simulink model "rx80211a3l"  (R2016a)
settings: Solver=FixedStepDiscrete  SolverMode=SingleTasking  StartTime=0.0  StopTime=46*tpf  RelTol=1e-3
PreLoadFcn:
  | [srx, str, ffv, stx, stb, spi, spl, spq, ntf, cdi, cds] = rx80211a_r0();
InitFcn:
  | if ~exist('srx','var')
  | [srx, str, ffv, stx, stb, spi, spl, spq, ntf, cdi, cds] = rx80211a_r0();
  | end
  | bitrate = 6e6; % 6 Mbits per second
  | crf = 2; % constant redundancy factor (from conv enc)
  | nepsc = 16; % #empty+pilot subcarriers
  | ncps = 16; % #cyclic prefix samples
  | ndbpf = 24; % #data bits per frame
  | ncbpf = ndbpf * crf; % #coded bits per frame
  | nscpf = ncbpf + nepsc; % #subcarriers per frame
  | nspf = nscpf + 16; % #samples per frame
  | tps = 1e-5; %tpf/nspf; % sample time
  | tpf = tps*nspf; %ndbpf/bitrate; % frame time
undefined symbols (not defined in the file): cds, ntf, srx
libraries: hdlsllib x34, simulink x17, dspxfrm3 x1, dspstat3 x1, commdigbbndpm3 x1, commcnvcod2 x1
settings Model: Creator=wchen  LastModifiedBy=bdroz
settings DataIOCC: LimitDataPoints=on  SaveFormat=Array  SaveOutput=off  SignalLogging=off  SaveTime=off
settings OptimizationCC: BlockReduction=off  ConditionallyExecuteInputs=off  DefaultParameterBehavior=Inlined  ExpressionDepthLimit=2147483647
settings DebuggingCC: AlgebraicLoopMsg=error  UnderspecifiedInitializationDetection=Classic  MergeDetectMultiDrivingBlocksExec=none  SolverPrmCheckMsg=warning  SingleTaskRateTransMsg=error  IntegerOverflowMsg=none  ParameterPrecisionLossMsg=none  AllowSymbolicDim=off  StateNameClashWarn=warning
settings HardwareCC: ProdBitPerPointer=32  ProdLargestAtomicFloat=None  ProdIntDivRoundTo=Undefined  ProdEndianess=Unspecified  ProdWordSize=32  ProdHWDeviceType=ASIC/FPGA->ASIC/FPGA  TargetBitPerPointer=64  TargetLongLongMode=on  TargetIntDivRoundTo=Zero  TargetEndianess=LittleEndian  TargetWordSize=64  TargetHWDeviceType=MATLAB Host  ProdEqTarget=off
settings ModelReferenceCC: PropagateSignalLabelsOutOfModel=off
settings ConfigComp: CovModelRefEnable=Off

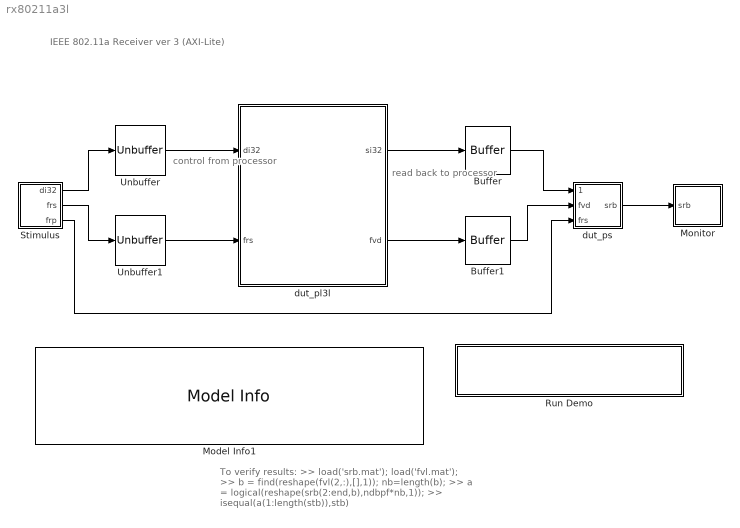
== system rx80211a3l ==
  note: control from
      | processor
  note: IEEE 802.11a Receiver ver 3 (AXI-Lite)
  note: read back to
      | processor
  note: To verify results:
      | >> load('srb.mat'); load('fvl.mat');
      | >> b = find(reshape(fvl(2,:),[],1)); nb=length(b);
      | >> a = logical(reshape(srb(2:end,b),ndbpf*nb,1));
      | >> isequal(a(1:length(stb)),stb)
  Buffer : Buffer  N=nspf  TreatMby1Signals=One channel  OutputFrames=off
  Buffer1 : Buffer  N=nspf  TreatMby1Signals=One channel  OutputFrames=off
  Model Info1 : simulink/Model-Wide Utilities/Model Info  Frame=on  DisplayStringWithTags=|  HorizontalTextAlignment=Left  LeftAlignmentValue=0.02  SourceBlockDiagram=rx80211a3l  TagMaxNumber=20
      | This example shows how to use HDL Workflow Advisor to 
      | generate a custom IP core which blink LEDs on FPGA board.
      | 
      | In MATLAB, type the following:
      |   hdladvisor('rx80211a3l/dut_pl3l')
  Monitor : Subsystem  TreatAsAtomicUnit=on
  Run Demo : Subsystem
      settings: OpenFcn=hdladvisor([bdroot, '/dut_pl'])
      mask Display: disp('Launch HDL Workflow Advisor')
  Stimulus : Subsystem
  Unbuffer : Unbuffer  SampleBasedProcessing=Same as frame based
  Unbuffer1 : Unbuffer  SampleBasedProcessing=Same as frame based
  dut_pl3l : Subsystem  TreatAsAtomicUnit=on
  dut_ps : Subsystem
  wires:
  Stimulus/1(di32) -> Unbuffer/1
  dut_pl3l/1(si32) -> Buffer/1
  Unbuffer/1 -> dut_pl3l/1(di32)
  Buffer/1 -> dut_ps/1(si32)
  dut_ps/1(srb) -> Monitor/1(srb)
  Stimulus/2(frs) -> Unbuffer1/1
  Unbuffer1/1 -> dut_pl3l/2(frs)
  dut_pl3l/2(fvd) -> Buffer1/1
  Buffer1/1 -> dut_ps/2(fvd)
  Stimulus/3(frp) -> dut_ps/3(frs)

== system rx80211a3l/Monitor ==
  srb : Inport
  Compare To Constant : simulink/Logic and Bit Operations/Compare To Constant  relop=>  const=uint16(0)  OutDataTypeStr=boolean
  Counter Free-Running : simulink/Sources/Counter Free-Running  NumBits=16  tsamp=tpf
  unpack_int32_into_bool24 : Subsystem
  write_srb_to_file1 : Subsystem
  wires:
  Counter Free-Running/1 -> Compare To Constant/1
  Compare To Constant/1 -> write_srb_to_file1/Enable
  unpack_int32_into_bool24/1(stx) -> write_srb_to_file1/1(srb)
  unpack_int32_into_bool24/2(fvd) -> write_srb_to_file1/2(fvl)
  srb/1 -> unpack_int32_into_bool24/1(di32)

== system rx80211a3l/Run Demo ==

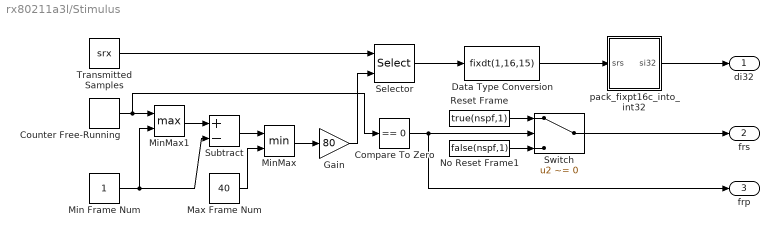
== system rx80211a3l/Stimulus ==
  Compare To Zero : simulink/Logic and Bit Operations/Compare To Zero  relop===  OutDataTypeStr=boolean
  Counter Free-Running : simulink/Sources/Counter Free-Running  NumBits=16  tsamp=tpf
  Data Type Conversion : DataTypeConversion  OutDataTypeStr=fixdt(1,16,15)
  Gain : Gain  Gain=80  OutDataTypeStr=uint16
  Max Frame Num : Constant  Value=40  OutDataTypeStr=uint16  SampleTime=tpf
  Min Frame Num : Constant  OutDataTypeStr=uint16  SampleTime=tpf
  MinMax : MinMax  Inputs=2
  MinMax1 : MinMax  Function=max  Inputs=2
  No Reset Frame1 : Constant  Value=false(nspf,1)  OutDataTypeStr=boolean  SampleTime=tpf
  Reset Frame : Constant  Value=true(nspf,1)  OutDataTypeStr=boolean  SampleTime=tpf
  Selector : Selector  IndexMode=Zero-based  InputPortWidth=3280  IndexOptions=Starting index (port)  Indices=[1 3]  OutputSizes=80
  Subtract : Sum  Inputs=+-
  Switch : Switch  Criteria=u2 ~= 0
  Transmitted Samples : Constant  Value=srx  SampleTime=tpf
  pack_fixpt16c_into_int32 : Subsystem
  di32 : Outport
  frs : Outport  Port=2
  frp : Outport  Port=3
  wires:
  Counter Free-Running/1 -> Compare To Zero/1, MinMax1/1
  Max Frame Num/1 -> MinMax/2
  MinMax/1 -> Gain/1
  Transmitted Samples/1 -> Selector/1
  Gain/1 -> Selector/2
  Selector/1 -> Data Type Conversion/1
  Data Type Conversion/1 -> pack_fixpt16c_into_int32/1(srs)
  pack_fixpt16c_into_int32/1(si32) -> di32/1
  Min Frame Num/1 -> MinMax1/2, Subtract/2
  Subtract/1 -> MinMax/1
  MinMax1/1 -> Subtract/1
  Compare To Zero/1 -> frp/1, Switch/2
  Switch/1 -> frs/1
  Reset Frame/1 -> Switch/1
  No Reset Frame1/1 -> Switch/3

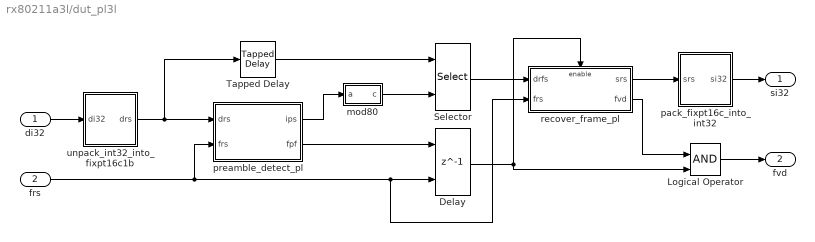
== system rx80211a3l/dut_pl3l ==
  di32 : Inport  OutDataTypeStr=uint32
  frs : Inport  Port=2  OutDataTypeStr=boolean
  Delay : Delay  DelayLength=1  InitialCondition=false  ExternalReset=Level  SampleTime=tps
      settings: InputPortMap=u0,r5
  Logical Operator : Logic  IconShape=distinctive  AllPortsSameDT=off  OutDataTypeStr=boolean
  Selector : Selector  IndexMode=Zero-based  InputPortWidth=80  IndexOptions=Starting index (port)  Indices=[1 3]  OutputSizes=1
  Tapped Delay : simulink/Discrete/Tapped Delay  vinit=complex(0.0)  samptime=tps  NumDelays=79  DelayOrder=Oldest  includeCurrent=on
  mod80 : Subsystem
  pack_fixpt16c_into_int32 : Subsystem
  preamble_detect_pl : Subsystem
  recover_frame_pl : Subsystem  TreatAsAtomicUnit=on
  unpack_int32_into_fixpt16c1b : Subsystem
  si32 : Outport
  fvd : Outport  Port=2
  wires:
  di32/1 -> unpack_int32_into_fixpt16c1b/1(di32)
  unpack_int32_into_fixpt16c1b/1(drs) -> Tapped Delay/1, preamble_detect_pl/1(drs)
  preamble_detect_pl/2(fpf) -> Delay/1
  recover_frame_pl/1(srs) -> pack_fixpt16c_into_int32/1(srs)
  Tapped Delay/1 -> Selector/1
  preamble_detect_pl/1(ips) -> mod80/1(a)
  Selector/1 -> recover_frame_pl/1(drfs)
  mod80/1(c) -> Selector/2
  Delay/1 -> recover_frame_pl/Enable, Logical Operator/2
  frs/1 -> preamble_detect_pl/2(frs), recover_frame_pl/2(frs), Delay/2
  pack_fixpt16c_into_int32/1(si32) -> si32/1
  Logical Operator/1 -> fvd/1
  recover_frame_pl/2(fvd) -> Logical Operator/1

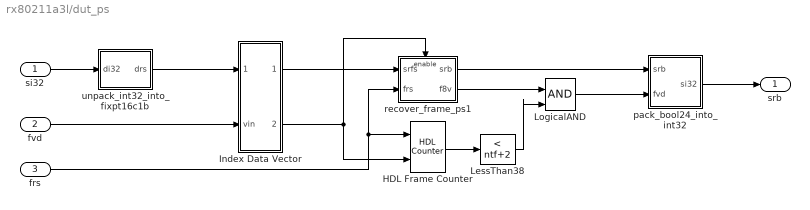
== system rx80211a3l/dut_ps ==
  si32 : Inport
  fvd : Inport  Port=2
  frs : Inport  Port=3
  HDL Frame Counter : hdlsllib/HDL Operations/HDL Counter  CountType=Free running  CountInit=0  CountStep=1  CountMax=25  CountFromType=Initial value  CountFrom=0  CountResetPort=on  CountLoadPort=off  CountEnbPort=on  CountDirPort=off  CountDataType=Unsigned  CountWordLen=8  CountFracLen=0  CountSampTime=1
  Index Data Vector : Subsystem
  LessThan38 : simulink/Logic and Bit Operations/Compare To Constant  relop=<  const=ntf+2  OutDataTypeStr=boolean
  LogicalAND : Logic  IconShape=distinctive  AllPortsSameDT=off  OutDataTypeStr=boolean
  pack_bool24_into_int32 : Subsystem
  recover_frame_ps1 : Subsystem  TreatAsAtomicUnit=on
  unpack_int32_into_fixpt16c1b : Subsystem
  srb : Outport
  wires:
  recover_frame_ps1/1(srb) -> pack_bool24_into_int32/1(srb)
  pack_bool24_into_int32/1(si32) -> srb/1
  frs/1 -> recover_frame_ps1/2(frs), HDL Frame Counter/1
  HDL Frame Counter/1 -> LessThan38/1
  LessThan38/1 -> LogicalAND/2
  LogicalAND/1 -> pack_bool24_into_int32/2(fvd)
  recover_frame_ps1/2(f8v) -> LogicalAND/1
  si32/1 -> unpack_int32_into_fixpt16c1b/1(di32)
  Index Data Vector/2(vout) -> recover_frame_ps1/Enable, HDL Frame Counter/2
  fvd/1 -> Index Data Vector/2(vin)
  unpack_int32_into_fixpt16c1b/1(drs) -> Index Data Vector/1(din)
  Index Data Vector/1(dout) -> recover_frame_ps1/1(srfs)

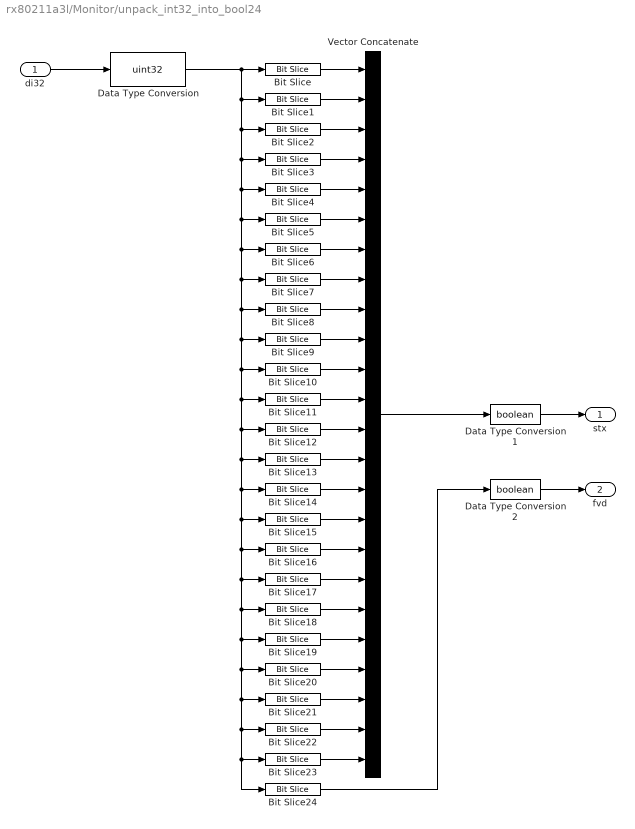
== system rx80211a3l/Monitor/unpack_int32_into_bool24 ==
  di32 : Inport
  Bit Slice : hdlsllib/HDL Operations/Bit Slice  lidx=31  ridx=31
      settings: AttributesFormatString=%<lidx>
  Bit Slice1 : hdlsllib/HDL Operations/Bit Slice  lidx=30  ridx=30
      settings: AttributesFormatString=%<lidx>
  Bit Slice10 : hdlsllib/HDL Operations/Bit Slice  lidx=21  ridx=21
      settings: AttributesFormatString=%<lidx>
  Bit Slice11 : hdlsllib/HDL Operations/Bit Slice  lidx=20  ridx=20
      settings: AttributesFormatString=%<lidx>
  Bit Slice12 : hdlsllib/HDL Operations/Bit Slice  lidx=19  ridx=19
      settings: AttributesFormatString=%<lidx>
  Bit Slice13 : hdlsllib/HDL Operations/Bit Slice  lidx=18  ridx=18
      settings: AttributesFormatString=%<lidx>
  Bit Slice14 : hdlsllib/HDL Operations/Bit Slice  lidx=17  ridx=17
      settings: AttributesFormatString=%<lidx>
  Bit Slice15 : hdlsllib/HDL Operations/Bit Slice  lidx=16  ridx=16
      settings: AttributesFormatString=%<lidx>
  Bit Slice16 : hdlsllib/HDL Operations/Bit Slice  lidx=15  ridx=15
      settings: AttributesFormatString=%<lidx>
  Bit Slice17 : hdlsllib/HDL Operations/Bit Slice  lidx=14  ridx=14
      settings: AttributesFormatString=%<lidx>
  Bit Slice18 : hdlsllib/HDL Operations/Bit Slice  lidx=13  ridx=13
      settings: AttributesFormatString=%<lidx>
  Bit Slice19 : hdlsllib/HDL Operations/Bit Slice  lidx=12  ridx=12
      settings: AttributesFormatString=%<lidx>
  Bit Slice2 : hdlsllib/HDL Operations/Bit Slice  lidx=29  ridx=29
      settings: AttributesFormatString=%<lidx>
  Bit Slice20 : hdlsllib/HDL Operations/Bit Slice  lidx=11  ridx=11
      settings: AttributesFormatString=%<lidx>
  Bit Slice21 : hdlsllib/HDL Operations/Bit Slice  lidx=10  ridx=10
      settings: AttributesFormatString=%<lidx>
  Bit Slice22 : hdlsllib/HDL Operations/Bit Slice  lidx=9  ridx=9
      settings: AttributesFormatString=%<lidx>
  Bit Slice23 : hdlsllib/HDL Operations/Bit Slice  lidx=8  ridx=8
      settings: AttributesFormatString=%<lidx>
  Bit Slice24 : hdlsllib/HDL Operations/Bit Slice  lidx=7  ridx=7
      settings: AttributesFormatString=%<lidx>
  Bit Slice3 : hdlsllib/HDL Operations/Bit Slice  lidx=28  ridx=28
      settings: AttributesFormatString=%<lidx>
  Bit Slice4 : hdlsllib/HDL Operations/Bit Slice  lidx=27  ridx=27
      settings: AttributesFormatString=%<lidx>
  Bit Slice5 : hdlsllib/HDL Operations/Bit Slice  lidx=26  ridx=26
      settings: AttributesFormatString=%<lidx>
  Bit Slice6 : hdlsllib/HDL Operations/Bit Slice  lidx=25  ridx=25
      settings: AttributesFormatString=%<lidx>
  Bit Slice7 : hdlsllib/HDL Operations/Bit Slice  lidx=24  ridx=24
      settings: AttributesFormatString=%<lidx>
  Bit Slice8 : hdlsllib/HDL Operations/Bit Slice  lidx=23  ridx=23
      settings: AttributesFormatString=%<lidx>
  Bit Slice9 : hdlsllib/HDL Operations/Bit Slice  lidx=22  ridx=22
      settings: AttributesFormatString=%<lidx>
  Data Type Conversion : DataTypeConversion  OutDataTypeStr=uint32  ConvertRealWorld=Stored Integer (SI)
  Data Type Conversion1 : DataTypeConversion  OutDataTypeStr=boolean
  Data Type Conversion2 : DataTypeConversion  OutDataTypeStr=boolean
  Vector Concatenate : Concatenate  NumInputs=24
  stx : Outport
  fvd : Outport  Port=2
  wires:
  di32/1 -> Data Type Conversion/1
  Vector Concatenate/1 -> Data Type Conversion1/1
  Bit Slice24/1 -> Data Type Conversion2/1
  Data Type Conversion/1 -> Bit Slice1/1, Bit Slice2/1, Bit Slice3/1, Bit Slice4/1, Bit Slice5/1, Bit Slice7/1, Bit Slice8/1, Bit Slice9/1, Bit Slice11/1, Bit Slice12/1, Bit Slice13/1, Bit Slice15/1, Bit Slice17/1, Bit Slice18/1, Bit Slice19/1, Bit Slice20/1, Bit Slice21/1, Bit Slice24/1, Bit Slice23/1, Bit Slice22/1, Bit Slice16/1, Bit Slice14/1, Bit Slice10/1, Bit Slice6/1, Bit Slice/1
  Bit Slice23/1 -> Vector Concatenate/24
  Bit Slice22/1 -> Vector Concatenate/23
  Bit Slice21/1 -> Vector Concatenate/22
  Bit Slice20/1 -> Vector Concatenate/21
  Bit Slice19/1 -> Vector Concatenate/20
  Bit Slice18/1 -> Vector Concatenate/19
  Bit Slice17/1 -> Vector Concatenate/18
  Bit Slice16/1 -> Vector Concatenate/17
  Bit Slice15/1 -> Vector Concatenate/16
  Bit Slice14/1 -> Vector Concatenate/15
  Bit Slice13/1 -> Vector Concatenate/14
  Bit Slice12/1 -> Vector Concatenate/13
  Bit Slice11/1 -> Vector Concatenate/12
  Bit Slice10/1 -> Vector Concatenate/11
  Bit Slice9/1 -> Vector Concatenate/10
  Bit Slice8/1 -> Vector Concatenate/9
  Bit Slice7/1 -> Vector Concatenate/8
  Bit Slice6/1 -> Vector Concatenate/7
  Bit Slice5/1 -> Vector Concatenate/6
  Bit Slice4/1 -> Vector Concatenate/5
  Bit Slice3/1 -> Vector Concatenate/4
  Bit Slice2/1 -> Vector Concatenate/3
  Bit Slice1/1 -> Vector Concatenate/2
  Bit Slice/1 -> Vector Concatenate/1
  Data Type Conversion1/1 -> stx/1
  Data Type Conversion2/1 -> fvd/1

== system rx80211a3l/Monitor/write_srb_to_file1 ==
  srb : Inport
  fvl : Inport  Port=2
  Enable : EnablePort
  Data Type Conversion : DataTypeConversion  OutDataTypeStr=double
  Data Type Conversion1 : DataTypeConversion  OutDataTypeStr=double
  To File : ToFile  Filename=srb.mat  MatrixName=srb  SampleTime=tpf
  To File1 : ToFile  Filename=fvl.mat  MatrixName=fvl  SampleTime=tpf
  wires:
  fvl/1 -> Data Type Conversion1/1
  Data Type Conversion1/1 -> To File1/1
  srb/1 -> Data Type Conversion/1
  Data Type Conversion/1 -> To File/1

== system rx80211a3l/Stimulus/pack_fixpt16c_into_int32 ==
  srs : Inport
  Bit Concat : hdlsllib/HDL Operations/Bit Concat  numInputs=2
  Complex to Real-Imag : ComplexToRealImag
  si32 : Outport
  wires:
  srs/1 -> Complex to Real-Imag/1
  Complex to Real-Imag/1 -> Bit Concat/1
  Bit Concat/1 -> si32/1
  Complex to Real-Imag/2 -> Bit Concat/2

== system rx80211a3l/dut_pl3l/mod80 ==
  a : Inport
  Constant80 : Constant  Value=uint8(80)  OutDataTypeStr=uint8  SampleTime=tps
  Divide : Product  Inputs=*/  SaturateOnIntegerOverflow=on  RndMeth=Zero
  Product : Product  OutDataTypeStr=uint8
  Subtract : Sum  Inputs=+-  OutDataTypeStr=uint8
  c : Outport
  wires:
  a/1 -> Subtract/1, Divide/1  "a"
  Constant80/1 -> Product/2, Divide/2  "b"
  Divide/1 -> Product/1
  Product/1 -> Subtract/2
  Subtract/1 -> c/1  "c"

== system rx80211a3l/dut_pl3l/pack_fixpt16c_into_int32 ==
  srs : Inport
  Bit Concat : hdlsllib/HDL Operations/Bit Concat  numInputs=2
  Complex to Real-Imag : ComplexToRealImag
  si32 : Outport
  wires:
  srs/1 -> Complex to Real-Imag/1
  Complex to Real-Imag/1 -> Bit Concat/1
  Bit Concat/1 -> si32/1
  Complex to Real-Imag/2 -> Bit Concat/2

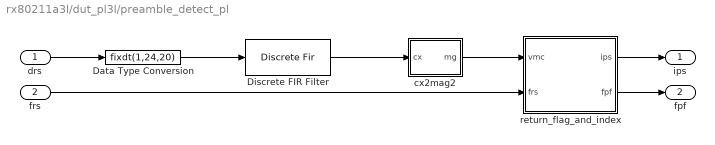
== system rx80211a3l/dut_pl3l/preamble_detect_pl ==
  drs : Inport
  frs : Inport  Port=2
  Data Type Conversion : DataTypeConversion  OutDataTypeStr=fixdt(1,24,20)
      settings: AttributesFormatString=%<OutDataTypeStr>
  Discrete FIR Filter : DiscreteFir  Coefficients=spl(end:-1:1)'  InitialStates=complex(0.0)  SampleTime=tps  CoefDataTypeStr=fixdt(1,24,20)  ProductDataTypeStr=fixdt(1,24,20)  AccumDataTypeStr=fixdt(1,24,20)  OutDataTypeStr=fixdt(1,24,20)
  cx2mag2 : Subsystem
  return_flag_and_index : Subsystem
  ips : Outport
  fpf : Outport  Port=2
  wires:
  return_flag_and_index/1(ips) -> ips/1
  return_flag_and_index/2(fpf) -> fpf/1
  cx2mag2/1(mg) -> return_flag_and_index/1(vmc)
  drs/1 -> Data Type Conversion/1
  Discrete FIR Filter/1 -> cx2mag2/1(cx)
  frs/1 -> return_flag_and_index/2(frs)
  Data Type Conversion/1 -> Discrete FIR Filter/1

== system rx80211a3l/dut_pl3l/recover_frame_pl ==
  drfs : Inport
  frs : Inport  Port=2
  Enable : EnablePort
  fft : Subsystem
  remove_cyclic_prefix : Subsystem
  srs : Outport  InitialOutput=0
  fvd : Outport  Port=2  InitialOutput=0
  wires:
  drfs/1 -> remove_cyclic_prefix/1(drfs)
  remove_cyclic_prefix/1(dcp) -> fft/1(dcp)
  frs/1 -> remove_cyclic_prefix/2(frs), fft/3(frs)
  remove_cyclic_prefix/2(fvo) -> fft/2(fvi)
  fft/1(dft) -> srs/1
  fft/2(fvo) -> fvd/1

== system rx80211a3l/dut_pl3l/unpack_int32_into_fixpt16c1b ==
  di32 : Inport
  Data Type Conversion : DataTypeConversion  OutDataTypeStr=fixdt(1,16,15)  ConvertRealWorld=Stored Integer (SI)
      settings: AttributesFormatString=%<OutDataTypeStr>
  Data Type Conversion1 : DataTypeConversion  OutDataTypeStr=fixdt(1,16,15)  ConvertRealWorld=Stored Integer (SI)
      settings: AttributesFormatString=%<OutDataTypeStr>
  Extract Bits : simulink/Logic and Bit Operations/Extract Bits  bitsToExtract=Upper half  numBits=8  bitIdxRange=[0 7]  outScalingMode=Preserve fixed-point scaling
  Extract Bits1 : simulink/Logic and Bit Operations/Extract Bits  bitsToExtract=Lower half  numBits=8  bitIdxRange=[0 7]  outScalingMode=Preserve fixed-point scaling
  Real-Imag to Complex : RealImagToComplex
  drs : Outport
  wires:
  di32/1 -> Extract Bits1/1, Extract Bits/1
  Extract Bits/1 -> Data Type Conversion/1
  Real-Imag to Complex/1 -> drs/1
  Extract Bits1/1 -> Data Type Conversion1/1
  Data Type Conversion/1 -> Real-Imag to Complex/1
  Data Type Conversion1/1 -> Real-Imag to Complex/2

== system rx80211a3l/dut_ps/Index Data Vector ==
  din : Inport
  vin : Inport  Port=2
  Maximum : dspstat3/Maximum  fcn=Value and Index  reset=None  InputProcessing=Columns as channels (frame based)  indexBase=Zero  operateOver=Each column  Dimension=1  operation=maximum  roiEnable=off  roiType=Rectangles  roiPortion=Entire ROI  roiOutput=Individual statistics for each ROI  roiFlag=off  accumDataTypeStr=Inherit: Same as product output  accumLastDataTypeStr=Inherit: Same as product output  roundingMode=Floor  overflowMode=off
  Selector : Selector  IndexMode=Zero-based  InputPortWidth=nspf  IndexOptions=Starting index (port)  Indices=0  OutputSizes=64
  Subsystem : Subsystem  Commented=on
  dout : Outport
  vout : Outport  Port=2
  wires:
  vin/1 -> Maximum/1
  din/1 -> Selector/1
  Selector/1 -> dout/1
  Maximum/2 -> Selector/2
  Maximum/1 -> vout/1

== system rx80211a3l/dut_ps/pack_bool24_into_int32 ==
  srb : Inport
  fvd : Inport  Port=2
  Bit Concat : hdlsllib/HDL Operations/Bit Concat  numInputs=1
  Constant 7 False Bits : Constant  Value=false(7,1)  OutDataTypeStr=boolean  SampleTime=tpf
  Data Type Conversion : DataTypeConversion  OutDataTypeStr=uint32  ConvertRealWorld=Stored Integer (SI)
  Vector Concatenate : Concatenate  NumInputs=3
  si32 : Outport
  wires:
  Vector Concatenate/1 -> Bit Concat/1
  srb/1 -> Vector Concatenate/1
  fvd/1 -> Vector Concatenate/2
  Constant 7 False Bits/1 -> Vector Concatenate/3
  Data Type Conversion/1 -> si32/1
  Bit Concat/1 -> Data Type Conversion/1

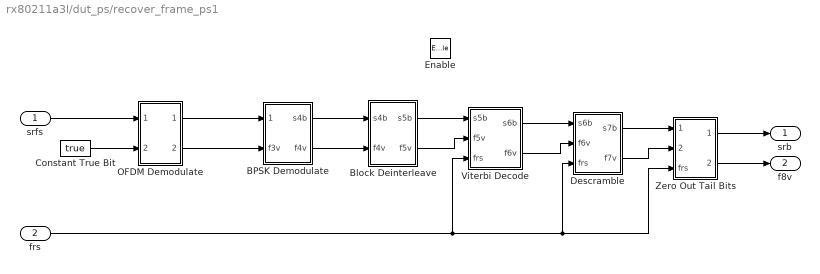
== system rx80211a3l/dut_ps/recover_frame_ps1 ==
  srfs : Inport
  frs : Inport  Port=2
  Enable : EnablePort
  BPSK Demodulate : Subsystem
  Block Deinterleave : Subsystem
  Constant True Bit : Constant  Value=true  OutDataTypeStr=boolean  SampleTime=tpf
  Descramble : Subsystem
  OFDM Demodulate : Subsystem
  Viterbi Decode : Subsystem
  Zero Out Tail Bits : Subsystem
  srb : Outport  InitialOutput=0
  f8v : Outport  Port=2  InitialOutput=0
  wires:
  frs/1 -> Descramble/3(frs), Zero Out Tail Bits/3(frs), Viterbi Decode/3(frs)
  OFDM Demodulate/1(d3m) -> BPSK Demodulate/1(d3m)
  BPSK Demodulate/1(s4b) -> Block Deinterleave/1(s4b)
  Block Deinterleave/1(s5b) -> Viterbi Decode/1(s5b)
  Viterbi Decode/1(s6b) -> Descramble/1(s6b)
  Descramble/1(s7b) -> Zero Out Tail Bits/1(s7b)
  Zero Out Tail Bits/1(s8b) -> srb/1
  Constant True Bit/1 -> OFDM Demodulate/2(f0v)
  OFDM Demodulate/2(f3v) -> BPSK Demodulate/2(f3v)
  BPSK Demodulate/2(f4v) -> Block Deinterleave/2(f4v)
  Block Deinterleave/2(f5v) -> Viterbi Decode/2(f5v)
  Viterbi Decode/2(f6v) -> Descramble/2(f6v)
  Descramble/2(f7v) -> Zero Out Tail Bits/2(f7v)
  Zero Out Tail Bits/2(f8v) -> f8v/1
  srfs/1 -> OFDM Demodulate/1(d0s)

== system rx80211a3l/dut_ps/unpack_int32_into_fixpt16c1b ==
  di32 : Inport
  Data Type Conversion : DataTypeConversion  OutDataTypeStr=fixdt(1,16,14)  ConvertRealWorld=Stored Integer (SI)
      settings: AttributesFormatString=%<OutDataTypeStr>
  Data Type Conversion1 : DataTypeConversion  OutDataTypeStr=fixdt(1,16,14)  ConvertRealWorld=Stored Integer (SI)
      settings: AttributesFormatString=%<OutDataTypeStr>
  Extract Bits : simulink/Logic and Bit Operations/Extract Bits  bitsToExtract=Upper half  numBits=8  bitIdxRange=[0 7]  outScalingMode=Preserve fixed-point scaling
  Extract Bits1 : simulink/Logic and Bit Operations/Extract Bits  bitsToExtract=Lower half  numBits=8  bitIdxRange=[0 7]  outScalingMode=Preserve fixed-point scaling
  Real-Imag to Complex : RealImagToComplex
  drs : Outport
  wires:
  di32/1 -> Extract Bits1/1, Extract Bits/1
  Extract Bits/1 -> Data Type Conversion/1
  Real-Imag to Complex/1 -> drs/1
  Extract Bits1/1 -> Data Type Conversion1/1
  Data Type Conversion/1 -> Real-Imag to Complex/1
  Data Type Conversion1/1 -> Real-Imag to Complex/2

== system rx80211a3l/dut_pl3l/preamble_detect_pl/cx2mag2 ==
  cx : Inport
  Add : Sum  OutDataTypeStr=fixdt(1,16,12)  SaturateOnIntegerOverflow=on  LockScale=on
  Complex to Real-Imag : ComplexToRealImag
  Product : Product  OutDataTypeStr=fixdt(1,16,12)  SaturateOnIntegerOverflow=on  LockScale=on
  Product1 : Product  OutDataTypeStr=fixdt(1,16,12)  SaturateOnIntegerOverflow=on  LockScale=on
  mg : Outport
  wires:
  cx/1 -> Complex to Real-Imag/1
  Complex to Real-Imag/1 -> Product/1, Product/2
  Complex to Real-Imag/2 -> Product1/2, Product1/1
  Product/1 -> Add/1
  Product1/1 -> Add/2
  Add/1 -> mg/1

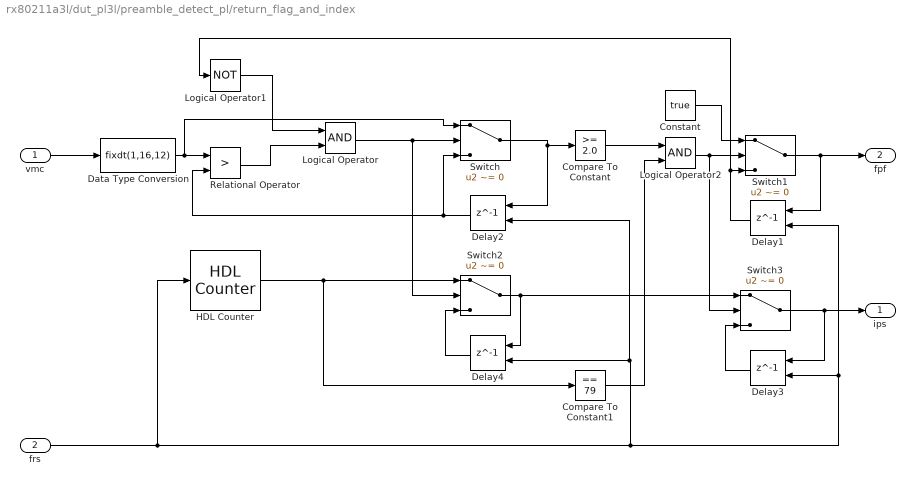
== system rx80211a3l/dut_pl3l/preamble_detect_pl/return_flag_and_index ==
  vmc : Inport
  frs : Inport  Port=2
  Compare To Constant : simulink/Logic and Bit Operations/Compare To Constant  relop=>=  const=2.0  OutDataTypeStr=boolean
  Compare To Constant1 : simulink/Logic and Bit Operations/Compare To Constant  relop===  const=79  OutDataTypeStr=boolean
  Constant : Constant  Value=true  OutDataTypeStr=boolean  SampleTime=tps
  Data Type Conversion : DataTypeConversion  OutDataTypeStr=fixdt(1,16,12)
  Delay1 : Delay  DelayLength=1  InitialCondition=false(1)  ExternalReset=Level  SampleTime=tps
      settings: InputPortMap=u0,r5
  Delay2 : Delay  DelayLength=1  ExternalReset=Level  SampleTime=tps
      settings: InputPortMap=u0,r5
  Delay3 : Delay  DelayLength=1  InitialCondition=uint8(0)  ExternalReset=Level  SampleTime=tps
      settings: InputPortMap=u0,r5
  Delay4 : Delay  DelayLength=1  InitialCondition=uint8(0)  ExternalReset=Level  SampleTime=tps
      settings: InputPortMap=u0,r5
  HDL Counter : hdlsllib/HDL Operations/HDL Counter  CountType=Count limited  CountInit=0  CountStep=1  CountMax=79  CountFromType=Initial value  CountFrom=0  CountResetPort=on  CountLoadPort=off  CountEnbPort=off  CountDirPort=off  CountDataType=Unsigned  CountWordLen=8  CountFracLen=0  CountSampTime=tps
  Logical Operator : Logic  AllPortsSameDT=off  OutDataTypeStr=boolean
  Logical Operator1 : Logic  Operator=NOT  AllPortsSameDT=off  OutDataTypeStr=boolean
  Logical Operator2 : Logic  AllPortsSameDT=off  OutDataTypeStr=boolean
  Relational Operator : RelationalOperator  Operator=>  OutDataTypeStr=boolean
  Switch : Switch  Criteria=u2 ~= 0  OutDataTypeStr=fixdt(1,16,12)
  Switch1 : Switch  Criteria=u2 ~= 0
  Switch2 : Switch  Criteria=u2 ~= 0  OutDataTypeStr=uint8
  Switch3 : Switch  Criteria=u2 ~= 0
  ips : Outport  OutDataTypeStr=uint8
  fpf : Outport  Port=2  OutDataTypeStr=boolean
  wires:
  Delay1/1 -> Switch1/3, Logical Operator1/1
  Switch/1 -> Delay2/1, Compare To Constant/1
  Compare To Constant/1 -> Logical Operator2/1
  Switch1/1 -> Delay1/1, fpf/1
  Constant/1 -> Switch1/1
  Switch3/1 -> Delay3/1, ips/1
  Delay2/1 -> Relational Operator/2, Switch/3
  vmc/1 -> Data Type Conversion/1
  Delay3/1 -> Switch3/3
  Relational Operator/1 -> Logical Operator/2
  Logical Operator1/1 -> Logical Operator/1
  Logical Operator/1 -> Switch2/2, Switch/2
  Logical Operator2/1 -> Switch3/2, Switch1/2
  Compare To Constant1/1 -> Logical Operator2/2
  HDL Counter/1 -> Compare To Constant1/1, Switch2/1
  Delay4/1 -> Switch2/3
  Data Type Conversion/1 -> Switch/1, Relational Operator/1
  Switch2/1 -> Switch3/1, Delay4/1
  frs/1 -> HDL Counter/1, Delay1/2, Delay3/2, Delay2/2, Delay4/2

== system rx80211a3l/dut_pl3l/recover_frame_pl/fft ==
  dcp : Inport
  fvi : Inport  Port=2
  frs : Inport  Port=3
  Data Type Conversion2 : DataTypeConversion  OutDataTypeStr=fixdt(1,16,14)  SaturateOnIntegerOverflow=on
      settings: AttributesFormatString=%<OutDataTypeStr>
  FFT HDL Optimized1 : dspxfrm3/FFT HDL Optimized  Architecture=Streaming Radix 2 (this choice will be removed -see release notes).  ComplexMultiplication=Use 4 multipliers and 2 adders  BitReversedOutput=off  Normalize=off  FFTLength=64  RoundingMethod=Floor  ResetInputPort=on  StartOutputPort=off  EndOutputPort=off  SimulateUsing=Code generation
  dft : Outport
  fvo : Outport  Port=2  OutDataTypeStr=boolean
  wires:
  FFT HDL Optimized1/1 -> Data Type Conversion2/1
  dcp/1 -> FFT HDL Optimized1/1
  fvi/1 -> FFT HDL Optimized1/2
  frs/1 -> FFT HDL Optimized1/3
  FFT HDL Optimized1/2 -> fvo/1
  Data Type Conversion2/1 -> dft/1

== system rx80211a3l/dut_pl3l/recover_frame_pl/remove_cyclic_prefix ==
  drfs : Inport
  frs : Inport  Port=2
  Compare To Constant : simulink/Logic and Bit Operations/Compare To Constant  relop=>  const=uint8(15)  OutDataTypeStr=boolean
  HDL Counter : hdlsllib/HDL Operations/HDL Counter  CountType=Count limited  CountInit=0  CountStep=1  CountMax=79  CountFromType=Initial value  CountFrom=0  CountResetPort=on  CountLoadPort=off  CountEnbPort=off  CountDirPort=off  CountDataType=Unsigned  CountWordLen=8  CountFracLen=0  CountSampTime=tps
  dcp : Outport
  fvo : Outport  Port=2
  wires:
  drfs/1 -> dcp/1
  HDL Counter/1 -> Compare To Constant/1
  frs/1 -> HDL Counter/1
  Compare To Constant/1 -> fvo/1

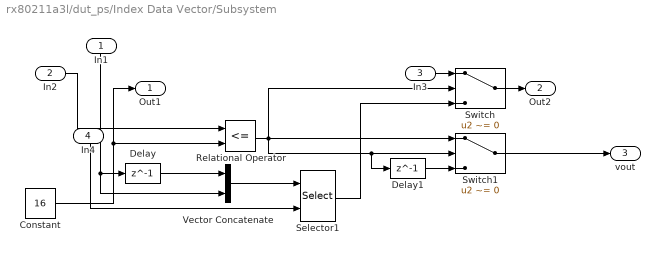
== system rx80211a3l/dut_ps/Index Data Vector/Subsystem ==
  In1 : Inport
  In2 : Inport  Port=2
  In3 : Inport  Port=3
  In4 : Inport  Port=4
  Constant : Constant  Value=16  OutDataTypeStr=uint8  SampleTime=tpf
  Delay : Delay  DelayLength=1  InitialCondition=complex(0.0)  SampleTime=tpf
  Delay1 : Delay  DelayLength=1  InitialCondition=false  SampleTime=tpf
  Relational Operator : RelationalOperator  Operator=<=  OutDataTypeStr=boolean
  Selector1 : Selector  IndexMode=Zero-based  InputPortWidth=2*nspf  IndexOptions=Starting index (port)  Indices=0  OutputSizes=64
  Switch : Switch  Criteria=u2 ~= 0
  Switch1 : Switch  Criteria=u2 ~= 0
  Vector Concatenate : Concatenate
  Out1 : Outport
  Out2 : Outport  Port=2
  vout : Outport  Port=3
  wires:
  Switch1/1 -> vout/1
  Relational Operator/1 -> Switch1/1, Delay1/1, Switch1/2, Switch/2
  Constant/1 -> Out1/1, Relational Operator/2
  Delay1/1 -> Switch1/3
  In2/1 -> Relational Operator/1
  In1/1 -> Vector Concatenate/2, Delay/1
  Vector Concatenate/1 -> Selector1/1
  Delay/1 -> Vector Concatenate/1
  Selector1/1 -> Switch/3
  Switch/1 -> Out2/1
  In4/1 -> Selector1/2
  In3/1 -> Switch/1

== system rx80211a3l/dut_ps/recover_frame_ps1/BPSK Demodulate ==
  d3m : Inport
  f3v : Inport  Port=2
  BPSK Demodulator Baseband : commdigbbndpm3/BPSK Demodulator Baseband  DecType=Hard decision  VarSource=Dialog  Variance=1  Ph=0  outDtype=boolean  derotateFactorWordLen=16  derotateFactorDataTypeStr=Inherit: Same word length as input  derotateFactorLastDataTypeStr=Inherit: Same word length as input
  Logical NOT : Logic  Operator=NOT  IconShape=distinctive  AllPortsSameDT=off  OutDataTypeStr=boolean
  s4b : Outport
  f4v : Outport  Port=2
  wires:
  d3m/1 -> BPSK Demodulator Baseband/1
  Logical NOT/1 -> s4b/1
  BPSK Demodulator Baseband/1 -> Logical NOT/1
  f3v/1 -> f4v/1

== system rx80211a3l/dut_ps/recover_frame_ps1/Block Deinterleave ==
  s4b : Inport
  f4v : Inport  Port=2
  block_deinterleave : Selector  IndexMode=Zero-based  InputPortWidth=48  IndexOptions=Index vector (dialog)  Indices=cdi  OutputSizes=1
  s5b : Outport
  f5v : Outport  Port=2
  wires:
  s4b/1 -> block_deinterleave/1
  block_deinterleave/1 -> s5b/1
  f4v/1 -> f5v/1

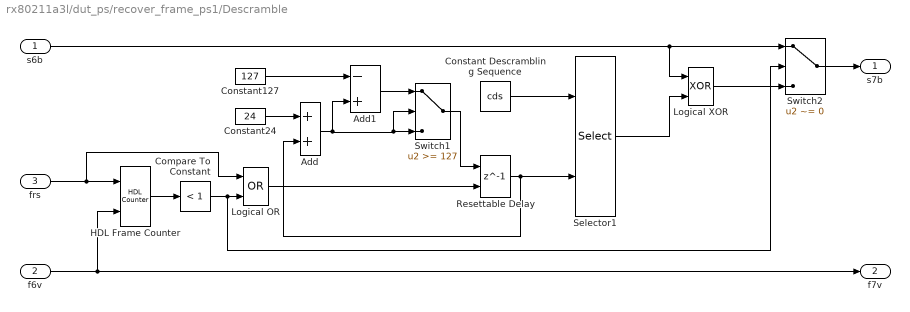
== system rx80211a3l/dut_ps/recover_frame_ps1/Descramble ==
  s6b : Inport
  f6v : Inport  Port=2
  frs : Inport  Port=3
  Add : Sum  OutDataTypeStr=uint8
  Add1 : Sum  Inputs=-+  OutDataTypeStr=uint8
  Compare To Constant : simulink/Logic and Bit Operations/Compare To Constant  relop=<  const=1  OutDataTypeStr=boolean
  Constant Descrambling Sequence : Constant  Value=cds  OutDataTypeStr=boolean  SampleTime=tpf
  Constant127 : Constant  Value=127  OutDataTypeStr=uint8  SampleTime=tpf
  Constant24 : Constant  Value=24  OutDataTypeStr=uint8  SampleTime=tpf
  HDL Frame Counter : hdlsllib/HDL Operations/HDL Counter  CountType=Free running  CountInit=0  CountStep=1  CountMax=23  CountFromType=Initial value  CountFrom=0  CountResetPort=on  CountLoadPort=off  CountEnbPort=on  CountDirPort=off  CountDataType=Unsigned  CountWordLen=16  CountFracLen=0  CountSampTime=tpf
  Logical OR : Logic  Operator=OR  IconShape=distinctive  AllPortsSameDT=off  OutDataTypeStr=boolean
  Logical XOR : Logic  Operator=XOR  IconShape=distinctive  AllPortsSameDT=off  OutDataTypeStr=boolean
  Resettable Delay : Delay  DelayLength=1  InitialCondition=uint8(0)  ExternalReset=Level  SampleTime=tpf
      settings: InputPortMap=u0,r5
  Selector1 : Selector  IndexMode=Zero-based  InputPortWidth=254  IndexOptions=Starting index (port)  Indices=[1 3]  OutputSizes=24
  Switch1 : Switch  Threshold=127
  Switch2 : Switch  Criteria=u2 ~= 0
  s7b : Outport
  f7v : Outport  Port=2
  wires:
  HDL Frame Counter/1 -> Compare To Constant/1
  f6v/1 -> HDL Frame Counter/2, f7v/1
  s6b/1 -> Switch2/1, Logical XOR/1
  frs/1 -> Logical OR/1, HDL Frame Counter/1
  Compare To Constant/1 -> Switch2/2, Logical OR/2
  Resettable Delay/1 -> Add/2, Selector1/2
  Constant Descrambling Sequence/1 -> Selector1/1
  Selector1/1 -> Logical XOR/2
  Constant24/1 -> Add/1
  Switch1/1 -> Resettable Delay/1
  Add/1 -> Add1/2, Switch1/2, Switch1/3
  Add1/1 -> Switch1/1
  Constant127/1 -> Add1/1
  Logical OR/1 -> Resettable Delay/2
  Logical XOR/1 -> Switch2/3
  Switch2/1 -> s7b/1

== system rx80211a3l/dut_ps/recover_frame_ps1/OFDM Demodulate ==
  d0s : Inport
  f0v : Inport  Port=2
  Subcarrier to Symbol Mapping : Selector  IndexMode=Zero-based  InputPortWidth=64  IndexOptions=Index vector (dialog)  Indices=[38:42, 44:56, 58:63, 1:6, 8:20, 22:26]  OutputSizes=1
  d3m : Outport
  f3v : Outport  Port=2
  wires:
  d0s/1 -> Subcarrier to Symbol Mapping/1  "d2s"
  Subcarrier to Symbol Mapping/1 -> d3m/1
  f0v/1 -> f3v/1

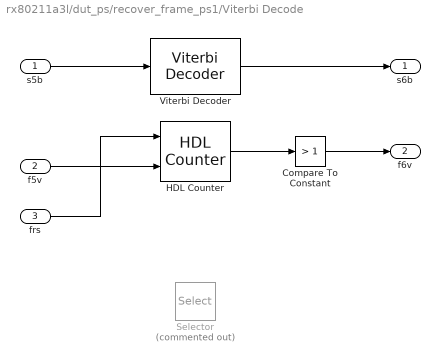
== system rx80211a3l/dut_ps/recover_frame_ps1/Viterbi Decode ==
  s5b : Inport
  f5v : Inport  Port=2
  frs : Inport  Port=3
  Compare To Constant : simulink/Logic and Bit Operations/Compare To Constant  relop=>  const=1  OutDataTypeStr=boolean
  HDL Counter : hdlsllib/HDL Operations/HDL Counter  CountType=Free running  CountInit=0  CountStep=1  CountMax=25  CountFromType=Initial value  CountFrom=0  CountResetPort=on  CountLoadPort=off  CountEnbPort=on  CountDirPort=off  CountDataType=Unsigned  CountWordLen=16  CountFracLen=0  CountSampTime=1
  Selector : Selector  Commented=on  IndexMode=Zero-based  InputPortWidth=48  IndexOptions=Starting index (dialog)  Indices=0  OutputSizes=24
  Viterbi Decoder : commcnvcod2/Viterbi Decoder  trellis=poly2trellis(7, [133,171])  isPunctured=off  punctureVector=[1; 1; 0; 1; 0; 1]  erasures=off  dectype=Hard decision  nsdecb=4  runSigValErrCheck=off  tbdepth=48  opmode=Continuous  reset=off  delayedResetAction=on  smWordLength=16  outDataType=boolean
  s6b : Outport
  f6v : Outport  Port=2
  wires:
  Viterbi Decoder/1 -> s6b/1
  s5b/1 -> Viterbi Decoder/1
  frs/1 -> HDL Counter/1
  f5v/1 -> HDL Counter/2
  HDL Counter/1 -> Compare To Constant/1
  Compare To Constant/1 -> f6v/1

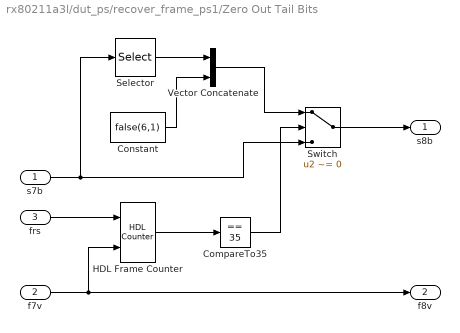
== system rx80211a3l/dut_ps/recover_frame_ps1/Zero Out Tail Bits ==
  s7b : Inport
  f7v : Inport  Port=2
  frs : Inport  Port=3
  CompareTo35 : simulink/Logic and Bit Operations/Compare To Constant  relop===  const=35  OutDataTypeStr=boolean
  Constant : Constant  Value=false(6,1)  OutDataTypeStr=boolean  SampleTime=tpf
  HDL Frame Counter : hdlsllib/HDL Operations/HDL Counter  CountType=Free running  CountInit=0  CountStep=1  CountMax=25  CountFromType=Initial value  CountFrom=0  CountResetPort=on  CountLoadPort=off  CountEnbPort=on  CountDirPort=off  CountDataType=Unsigned  CountWordLen=16  CountFracLen=0  CountSampTime=tpf
  Selector : Selector  IndexMode=Zero-based  InputPortWidth=24  IndexOptions=Index vector (dialog)  Indices=0:17  OutputSizes=1
  Switch : Switch  Criteria=u2 ~= 0  Threshold=36
  Vector Concatenate : Concatenate
  s8b : Outport
  f8v : Outport  Port=2
  wires:
  HDL Frame Counter/1 -> CompareTo35/1
  Vector Concatenate/1 -> Switch/1
  Switch/1 -> s8b/1
  s7b/1 -> Selector/1, Switch/3
  Constant/1 -> Vector Concatenate/2
  Selector/1 -> Vector Concatenate/1
  frs/1 -> HDL Frame Counter/1
  f7v/1 -> HDL Frame Counter/2, f8v/1
  CompareTo35/1 -> Switch/2
